simulink model "PID_Throttle"  (R2019b)
settings: Solver=FixedStepDiscrete  StartTime=0.0  StopTime=10.0  RelTol=1e-3
PreLoadFcn:
  | DLRNLPD =1
  | DLRIAMAXA = 1
  | CWDKNOLU = 1
  | DANTGESWNV = 1
  | DLRKPONLP0 = 1
  | DLRKPONLP3 = 1
  | CWDKNOLU = 1
  | DANTGESWNV = 1
  | DLRKPONLP0 = 1
  | DLRKDONLP0 = 1
  | DLRKPUNLP3 = 1
  | DANTSCHWNV = 1
  | DLRUMABAND = 1
  | DLRKDUNLP3 = 1
  | DLRUMAIINI = 1
undefined symbols (not defined in the file): DLRHAFTMN, DLRININI, DLRKREIS
libraries: simulink x3
settings Model: Creator=Guest-Pasand  LastModifiedBy=Guest-Pasand
settings OptimizationCC: DefaultParameterBehavior=Inlined  UseDivisionForNetSlopeComputation=on  GainParamInheritBuiltInType=on  UseFloatMulNetSlope=on  InlineInvariantSignals=on  PassReuseOutputArgsAs=Individual arguments  ZeroExternalMemoryAtStartup=off  ZeroInternalMemoryAtStartup=off  NoFixptDivByZeroProtection=on  EfficientFloat2IntCast=on  LifeSpan=1  OptimizeBlockOrder=speed  DifferentSizesBufferReuse=on  EfficientTunableParamExpr=on
settings DebuggingCC: ParameterTunabilityLossMsg=error
settings HardwareCC: ProdBitPerPointer=32  ProdBitPerSizeT=32  ProdBitPerPtrDiffT=32  ProdLargestAtomicInteger=Long  ProdLargestAtomicFloat=Double  ProdWordSize=32  ProdLongLongMode=on  ProdHWDeviceType=ARM Compatible->ARM Cortex
settings SFSimCC: MATLABDynamicMemAlloc=off
settings RTWCC: SystemTargetFile=ert.tlc  GenCodeOnly=on  TemplateMakefile=ert_default_tmf  GenerateReport=on  IncludeHyperlinkInReport=on  LaunchReport=on  GenerateTraceInfo=on  GenerateTraceReport=on  GenerateTraceReportSl=on  GenerateTraceReportSf=on  GenerateTraceReportEml=on  GenerateCodeMetricsReport=on
settings CodeAppCC: ForceParamTrailComments=on  IgnoreCustomStorageClasses=off  OperatorAnnotations=on  SimulinkDataObjDesc=on  SFDataObjDesc=on  CustomSymbolStrGlobalVar=rt$N$M  CustomSymbolStrType=$N$M  CustomSymbolStrFcn=$N$M$F  CustomSymbolStrMacro=$N$M  InsertBlockDesc=on
settings ERTTargetCC: TargetLangStandard=C99 (ISO)  GenerateSampleERTMain=on  IncludeMdlTerminateFcn=off  CombineSignalStateStructs=on  SuppressErrorStatus=on  SupportAbsoluteTime=off  SupportComplex=off  InlinedParameterPlacement=NonHierarchical  ERTCustomFileTemplate=example_file_process.tlc  ERTFilePackagingFormat=CompactWithDataFile

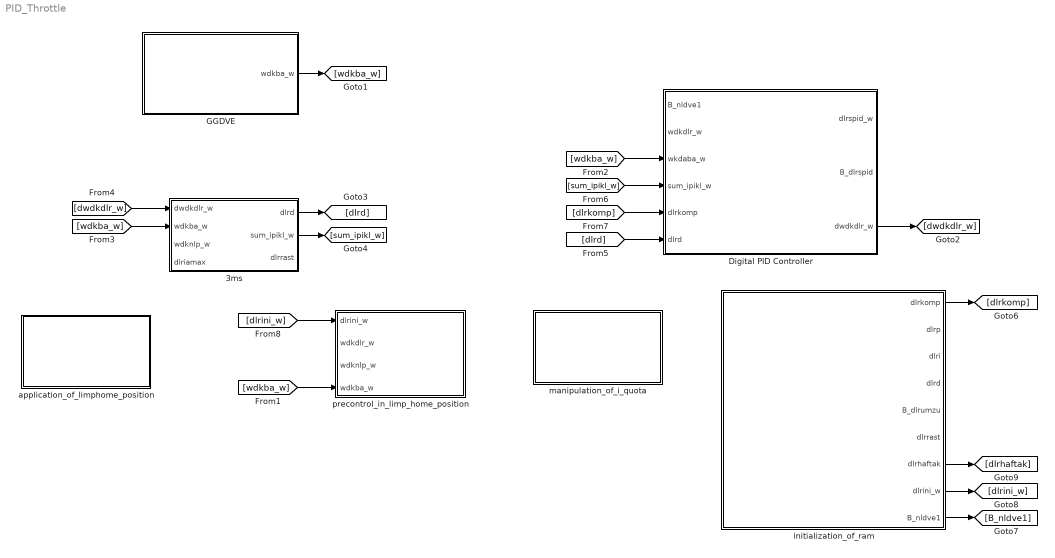
== system PID_Throttle ==
  3ms : Subsystem
  Digital PID Controller : Subsystem
  GGDVE : Subsystem
  application_of_limphome_position : Subsystem
  initialization_of_ram : Subsystem
  "manipulation_of_i_quota " : Subsystem
  precontrol_in_limp_home_position : Subsystem
  wires:
  GGDVE/1(wdkba_w) -> [wdkba_w]
  [wdkba_w] -> precontrol_in_limp_home_position/4(wdkba_w)
  [wdkba_w] -> Digital PID Controller/3(wkdaba_w)
  [wdkba_w] -> 3ms/2(wdkba_w)
  Digital PID Controller/3("dwdkdlr_w ") -> [dwdkdlr_w]
  [dwdkdlr_w] -> 3ms/1(dwdkdlr_w)
  3ms/1(dlrd) -> [dlrd]
  [dlrd] -> Digital PID Controller/6(dlrd)
  [sum_ipikl_w] -> Digital PID Controller/4(sum_ipikl_w)
  3ms/2(sum_ipikl_w) -> [sum_ipikl_w]
  initialization_of_ram/1(dlrkomp) -> [dlrkomp]
  [dlrkomp] -> Digital PID Controller/5(dlrkomp)
  initialization_of_ram/9(B_nldve1) -> [B_nldve1]
  initialization_of_ram/8(dlrini_w) -> [dlrini_w]
  initialization_of_ram/7("dlrhaftak ") -> [dlrhaftak]
  [dlrini_w] -> precontrol_in_limp_home_position/1(dlrini_w)

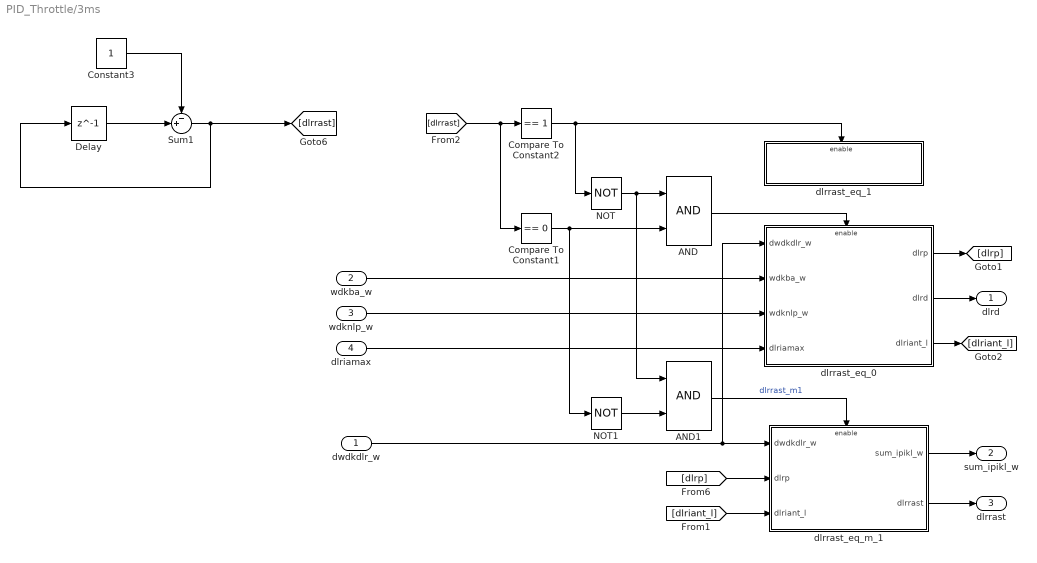
== system PID_Throttle/3ms ==
  dwdkdlr_w : Inport
  wdkba_w : Inport  Port=2
  wdknlp_w : Inport  Port=3
  dlriamax : Inport  Port=4
  AND : Logic  AllPortsSameDT=off  OutDataTypeStr=boolean
  AND1 : Logic  AllPortsSameDT=off  OutDataTypeStr=boolean
  Compare To Constant1 : simulink/Logic and Bit Operations/Compare To Constant  relop===  const=0  OutDataTypeStr=boolean
  Compare To Constant2 : simulink/Logic and Bit Operations/Compare To Constant  relop===  const=1  OutDataTypeStr=boolean
  Constant3 : Constant  VectorParams1D=off  OutDataTypeStr=int8
  Delay : Delay  DelayLength=1  InitialCondition=0
  NOT : Logic  Operator=NOT  IconShape=distinctive  AllPortsSameDT=off  OutDataTypeStr=boolean
  NOT1 : Logic  Operator=NOT  IconShape=distinctive  AllPortsSameDT=off  OutDataTypeStr=boolean
  Sum1 : Sum  Inputs=-+|
  dlrrast_eq_0 : Subsystem
  dlrrast_eq_1 : Subsystem
  dlrrast_eq_m_1 : Subsystem
  dlrd : Outport
  sum_ipikl_w : Outport  Port=2
  dlrrast : Outport  Port=3
  wires:
  Sum1/1 -> Delay/1, [dlrrast]
  Delay/1 -> Sum1/2
  Constant3/1 -> Sum1/1
  Compare To Constant1/1 -> NOT1/1, AND/2
  [dlrrast] -> Compare To Constant1/1, Compare To Constant2/1
  dlrrast_eq_0/1(dlrp) -> [dlrp]
  Compare To Constant2/1 -> dlrrast_eq_1/Enable, NOT/1
  AND/1 -> dlrrast_eq_0/Enable
  NOT/1 -> AND1/1, AND/1
  NOT1/1 -> AND1/2
  AND1/1 -> dlrrast_eq_m_1/Enable  "dlrrast_m1"
  [dlrp] -> dlrrast_eq_m_1/2(dlrp)
  dlrrast_eq_0/3(dlriant_l) -> [dlriant_l]
  [dlriant_l] -> dlrrast_eq_m_1/3(dlriant_l)
  dwdkdlr_w/1 -> dlrrast_eq_m_1/1(dwdkdlr_w), dlrrast_eq_0/1(dwdkdlr_w)
  wdkba_w/1 -> dlrrast_eq_0/2(wdkba_w)
  wdknlp_w/1 -> dlrrast_eq_0/3(wdknlp_w)
  dlrrast_eq_0/2(dlrd) -> dlrd/1
  dlriamax/1 -> dlrrast_eq_0/4(dlriamax)
  dlrrast_eq_m_1/1(sum_ipikl_w) -> sum_ipikl_w/1
  dlrrast_eq_m_1/2(dlrrast) -> dlrrast/1

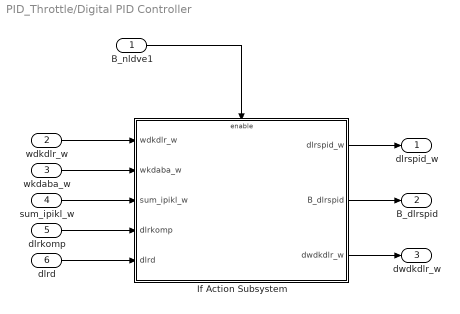
== system PID_Throttle/Digital PID Controller ==
  B_nldve1 : Inport  OutDataTypeStr=boolean
  wdkdlr_w : Inport  Port=2
  wkdaba_w : Inport  Port=3
  sum_ipikl_w : Inport  Port=4
  dlrkomp : Inport  Port=5
  dlrd : Inport  Port=6
  If Action Subsystem : Subsystem  TreatAsAtomicUnit=on
  dlrspid_w : Outport
  B_dlrspid : Outport  Port=2
  "dwdkdlr_w " : Outport  Port=3
  wires:
  wdkdlr_w/1 -> If Action Subsystem/1(wdkdlr_w)
  If Action Subsystem/1(dlrspid_w) -> dlrspid_w/1
  If Action Subsystem/2(B_dlrspid) -> B_dlrspid/1
  B_nldve1/1 -> If Action Subsystem/Enable
  dlrd/1 -> If Action Subsystem/5("dlrd ")
  dlrkomp/1 -> If Action Subsystem/4(dlrkomp)
  sum_ipikl_w/1 -> If Action Subsystem/3(sum_ipikl_w)
  wkdaba_w/1 -> If Action Subsystem/2(wkdaba_w)
  If Action Subsystem/3(dwdkdlr_w) -> "dwdkdlr_w "/1

== system PID_Throttle/GGDVE ==
  wdkba_w : Outport

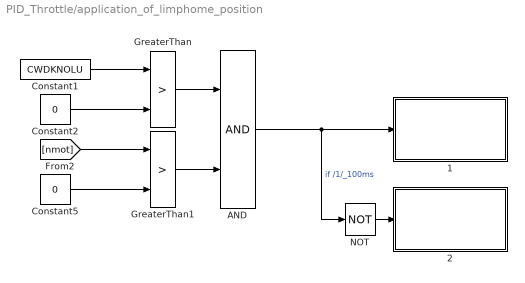
== system PID_Throttle/application_of_limphome_position ==
  1 : Subsystem
  2 : Subsystem
  AND : Logic  AllPortsSameDT=off  OutDataTypeStr=boolean
  Constant1 : Constant  Value=CWDKNOLU  VectorParams1D=off  OutDataTypeStr=int8
  Constant2 : Constant  Value=0  VectorParams1D=off  OutDataTypeStr=int8
  Constant5 : Constant  Value=0  VectorParams1D=off  OutDataTypeStr=int8
  GreaterThan : RelationalOperator  Operator=>  OutDataTypeStr=boolean  RndMeth=Simplest
  GreaterThan1 : RelationalOperator  Operator=>  OutDataTypeStr=boolean  RndMeth=Simplest
  NOT : Logic  Operator=NOT  IconShape=distinctive  AllPortsSameDT=off  OutDataTypeStr=boolean
  wires:
  Constant1/1 -> GreaterThan/1
  Constant2/1 -> GreaterThan/2
  Constant5/1 -> GreaterThan1/2
  [nmot] -> GreaterThan1/1
  GreaterThan/1 -> AND/1
  GreaterThan1/1 -> AND/2
  AND/1 -> NOT/1, 1/Enable  "if /1/_100ms"
  NOT/1 -> 2/Enable

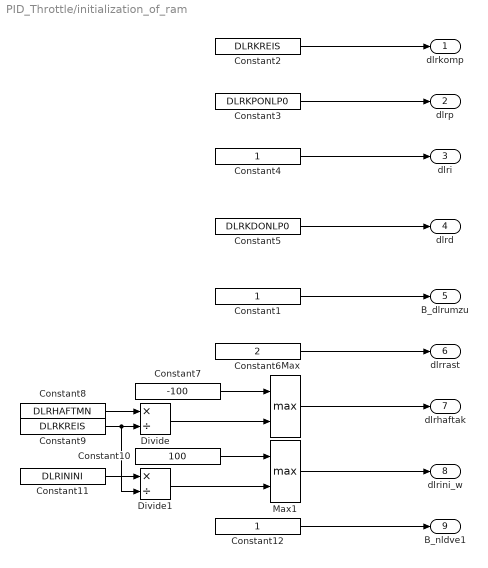
== system PID_Throttle/initialization_of_ram ==
  Constant1 : Constant  VectorParams1D=off
  Constant10 : Constant  Value=100  VectorParams1D=off
  Constant11 : Constant  Value=DLRININI  VectorParams1D=off
  Constant12 : Constant  VectorParams1D=off
  Constant2 : Constant  Value=DLRKREIS  VectorParams1D=off
  Constant3 : Constant  Value=DLRKPONLP0  VectorParams1D=off
  Constant4 : Constant  VectorParams1D=off
  Constant5 : Constant  Value=DLRKDONLP0  VectorParams1D=off
  Constant6 : Constant  Value=2  VectorParams1D=off
  Constant7 : Constant  Value=-100  VectorParams1D=off
  Constant8 : Constant  Value=DLRHAFTMN  VectorParams1D=off
  Constant9 : Constant  Value=DLRKREIS  VectorParams1D=off
  Divide : Product  Inputs=*/
  Divide1 : Product  Inputs=*/
  Max : MinMax  Function=max  Inputs=2
  Max1 : MinMax  Function=max  Inputs=2
  dlrkomp : Outport
  dlrp : Outport  Port=2
  "dlri " : Outport  Port=3
  dlrd : Outport  Port=4
  "B_dlrumzu " : Outport  Port=5
  dlrrast : Outport  Port=6
  "dlrhaftak " : Outport  Port=7
  dlrini_w : Outport  Port=8
  B_nldve1 : Outport  Port=9
  wires:
  Constant2/1 -> dlrkomp/1
  Constant3/1 -> dlrp/1
  Constant4/1 -> "dlri "/1
  Constant5/1 -> dlrd/1
  Constant1/1 -> "B_dlrumzu "/1
  Constant6/1 -> dlrrast/1
  Constant7/1 -> Max/1
  Constant8/1 -> Divide/1
  Divide/1 -> Max/2
  Divide1/1 -> Max1/2
  Constant9/1 -> Divide1/2, Divide/2
  Constant11/1 -> Divide1/1
  Constant10/1 -> Max1/1
  Max/1 -> "dlrhaftak "/1
  Max1/1 -> dlrini_w/1
  Constant12/1 -> B_nldve1/1

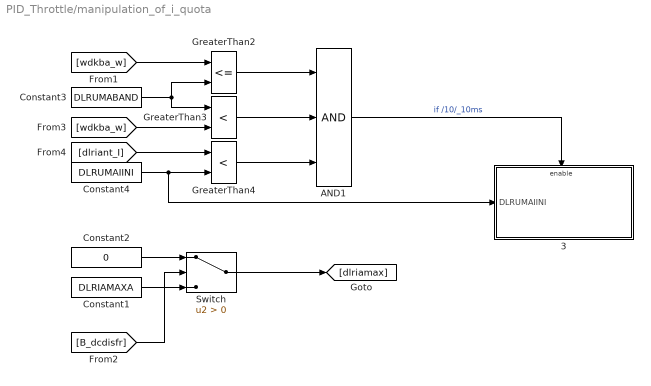
== system PID_Throttle/manipulation_of_i_quota  ==
  3 : Subsystem
  AND1 : Logic  Inputs=3  AllPortsSameDT=off  OutDataTypeStr=boolean
  Constant1 : Constant  Value=DLRIAMAXA  VectorParams1D=off  OutDataTypeStr=int8
  Constant2 : Constant  Value=0  VectorParams1D=off  OutDataTypeStr=int8
  Constant3 : Constant  Value=DLRUMABAND  VectorParams1D=off  OutDataTypeStr=int8
  Constant4 : Constant  Value=DLRUMAIINI  VectorParams1D=off  OutDataTypeStr=int8
  GreaterThan2 : RelationalOperator  Operator=<=  OutDataTypeStr=boolean  RndMeth=Simplest
  GreaterThan3 : RelationalOperator  Operator=<  OutDataTypeStr=boolean  RndMeth=Simplest
  GreaterThan4 : RelationalOperator  Operator=<  OutDataTypeStr=boolean  RndMeth=Simplest
  Switch : Switch  Criteria=u2 > Threshold
  wires:
  [wdkba_w] -> GreaterThan2/1
  Constant3/1 -> GreaterThan2/2, GreaterThan3/1
  [wdkba_w] -> GreaterThan3/2
  [dlriant_I] -> GreaterThan4/1
  Constant4/1 -> 3/1("DLRUMAIINI "), GreaterThan4/2
  GreaterThan4/1 -> AND1/3
  GreaterThan3/1 -> AND1/2
  GreaterThan2/1 -> AND1/1
  AND1/1 -> 3/Enable  "if /10/_10ms"
  Constant2/1 -> Switch/1
  Constant1/1 -> Switch/3
  [B_dcdisfr] -> Switch/2
  Switch/1 -> [dlriamax]

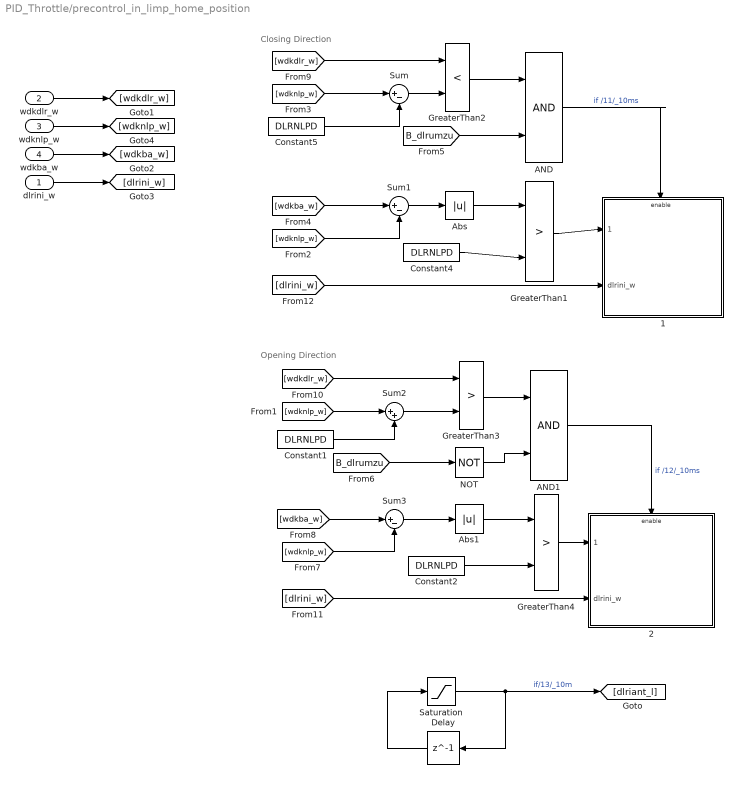
== system PID_Throttle/precontrol_in_limp_home_position ==
  note: Closing Direction
  note: Opening Direction
  dlrini_w : Inport
  wdkdlr_w : Inport  Port=2
  wdknlp_w : Inport  Port=3
  wdkba_w : Inport  Port=4
  1 : Subsystem
  2 : Subsystem
  AND : Logic  AllPortsSameDT=off  OutDataTypeStr=boolean
  AND1 : Logic  AllPortsSameDT=off  OutDataTypeStr=boolean
  Abs : Abs
  Abs1 : Abs
  Constant{1..2,4..5} (4 alike) : Constant  Value=DLRNLPD  VectorParams1D=off  OutDataTypeStr=int8
  Delay : Delay  DelayLength=1
  GreaterThan1 : RelationalOperator  Operator=>  OutDataTypeStr=boolean  RndMeth=Simplest
  GreaterThan2 : RelationalOperator  Operator=<  OutDataTypeStr=boolean  RndMeth=Simplest
  GreaterThan3 : RelationalOperator  Operator=>  OutDataTypeStr=boolean  RndMeth=Simplest
  GreaterThan4 : RelationalOperator  Operator=>  OutDataTypeStr=boolean  RndMeth=Simplest
  NOT : Logic  Operator=NOT  IconShape=distinctive  AllPortsSameDT=off  OutDataTypeStr=boolean
  Saturation : Saturate  UpperLimit=100  LowerLimit=-100
  Sum : Sum  Inputs=|+-
  Sum1 : Sum  Inputs=|+-
  Sum2 : Sum  Inputs=|++
  Sum3 : Sum  Inputs=|+-
  wires:
  Constant5/1 -> Sum/2
  Delay/1 -> Saturation/1
  GreaterThan3/1 -> AND1/1
  [wdkba_w] -> Sum3/1
  Sum3/1 -> Abs1/1
  GreaterThan4/1 -> 2/1(" ")
  Saturation/1 -> [dlriant_l], Delay/1  "if/13/_10m"
  Sum1/1 -> Abs/1
  AND1/1 -> 2/Enable  "if /12/_10ms"
  [wdknlp_w] -> Sum3/2
  Constant2/1 -> GreaterThan4/2
  Abs1/1 -> GreaterThan4/1
  [wdknlp_w] -> Sum2/1
  Constant1/1 -> Sum2/2
  NOT/1 -> AND1/2
  [wdknlp_w] -> Sum1/2
  Sum2/1 -> GreaterThan3/2
  [B_dlrumzu] -> NOT/1
  [wdkba_w] -> Sum1/1
  Sum/1 -> GreaterThan2/2
  Constant4/1 -> GreaterThan1/2
  [wdknlp_w] -> Sum/1
  AND/1 -> 1/Enable  "if /11/_10ms"
  GreaterThan1/1 -> 1/1(" ")
  Abs/1 -> GreaterThan1/1
  [B_dlrumzu] -> AND/2
  GreaterThan2/1 -> AND/1
  wdknlp_w/1 -> [wdknlp_w]
  wdkdlr_w/1 -> [wdkdlr_w]
  wdkba_w/1 -> [wdkba_w]
  [wdkdlr_w] -> GreaterThan2/1
  [wdkdlr_w] -> GreaterThan3/1
  dlrini_w/1 -> [dlrini_w]
  [dlrini_w] -> 2/2(dlrini_w)
  [dlrini_w] -> 1/2(dlrini_w)

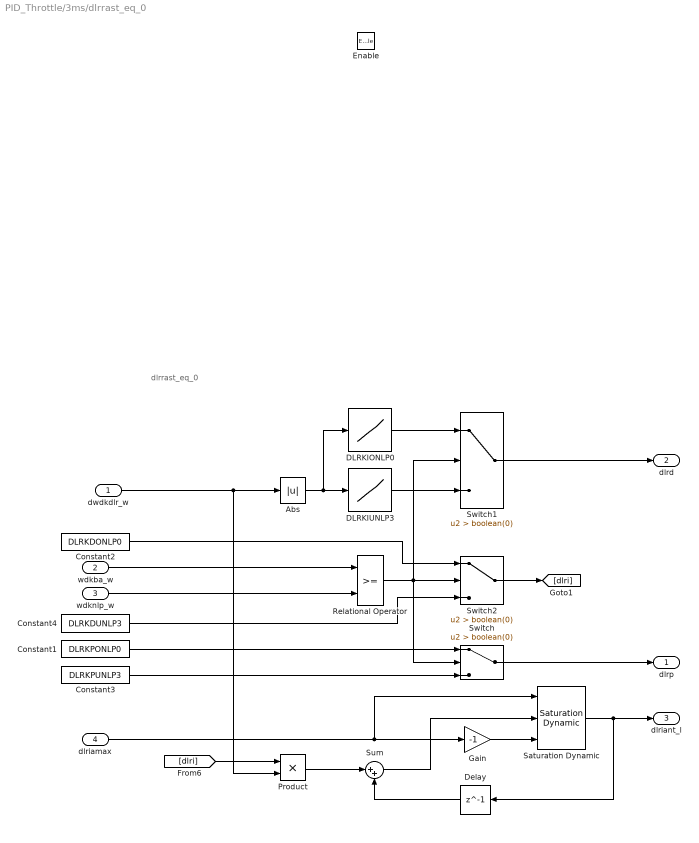
== system PID_Throttle/3ms/dlrrast_eq_0 ==
  note: dlrrast_eq_0
  dwdkdlr_w : Inport
  wdkba_w : Inport  Port=2
  wdknlp_w : Inport  Port=3
  dlriamax : Inport  Port=4
  Enable : EnablePort
  Abs : Abs  ZeroCross=off
  Constant1 : Constant  Value=DLRKPONLP0  VectorParams1D=off  OutDataTypeStr=int8
  Constant2 : Constant  Value=DLRKDONLP0  VectorParams1D=off  OutDataTypeStr=int8
  Constant3 : Constant  Value=DLRKPUNLP3  VectorParams1D=off  OutDataTypeStr=int8
  Constant4 : Constant  Value=DLRKDUNLP3  VectorParams1D=off  OutDataTypeStr=int8
  DLRKIONLP0 : Lookup_n-D  NumberOfTableDimensions=1  BreakpointsForDimension1=[-5:5]  Table=tanh([-5:5])  InternalRulePriority=Speed  RndMeth=Simplest  InputSameDT=on
  DLRKIUNLP3 : Lookup_n-D  NumberOfTableDimensions=1  BreakpointsForDimension1=[-5:5]  Table=tanh([-5:5])  InternalRulePriority=Speed  RndMeth=Simplest  InputSameDT=on
  Delay : Delay  DelayLength=1  InitialCondition=0
  Gain : Gain  Gain=-1  ParamDataTypeStr=double
  Product : Product
  Relational Operator : RelationalOperator  OutDataTypeStr=boolean  RndMeth=Simplest
  Saturation Dynamic : simulink/Discontinuities/Saturation Dynamic  OutMin=[]  OutMax=[]  OutDataTypeStr=Inherit: Same as second input  OutDataType=fixdt(1, 16)  OutScaling=2^-10  DoSatur=off
  Sum : Sum  Inputs=|++
  Switch : Switch  Criteria=u2 > Threshold  Threshold=boolean(0)
  Switch1 : Switch  Criteria=u2 > Threshold  Threshold=boolean(0)
  Switch2 : Switch  Criteria=u2 > Threshold  Threshold=boolean(0)
  dlrp : Outport
  dlrd : Outport  Port=2
  dlriant_l : Outport  Port=3
  wires:
  Switch1/1 -> dlrd/1
  Switch/1 -> dlrp/1
  Saturation Dynamic/1 -> dlriant_l/1, Delay/1
  Constant4/1 -> Switch2/3
  Constant1/1 -> Switch/1
  Constant3/1 -> Switch/3
  Constant2/1 -> Switch2/1
  wdknlp_w/1 -> Relational Operator/2
  Gain/1 -> Saturation Dynamic/3
  Abs/1 -> DLRKIUNLP3/1, DLRKIONLP0/1
  Delay/1 -> Sum/2
  Product/1 -> Sum/1
  Sum/1 -> Saturation Dynamic/2
  dlriamax/1 -> Saturation Dynamic/1, Gain/1
  [dlri] -> Product/1
  DLRKIUNLP3/1 -> Switch1/3
  wdkba_w/1 -> Relational Operator/1
  dwdkdlr_w/1 -> Product/2, Abs/1
  Relational Operator/1 -> Switch1/2, Switch2/2, Switch/2
  DLRKIONLP0/1 -> Switch1/1
  Switch2/1 -> [dlri]

== system PID_Throttle/3ms/dlrrast_eq_1 ==
  Enable : EnablePort

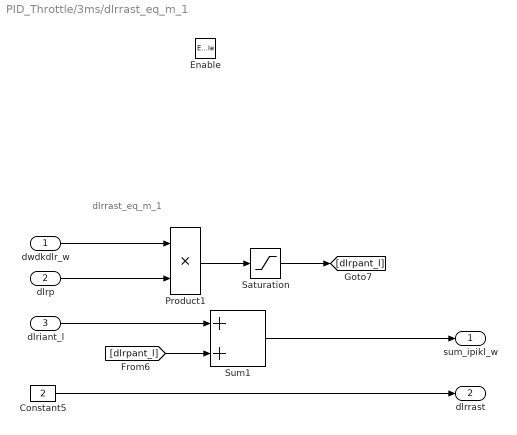
== system PID_Throttle/3ms/dlrrast_eq_m_1 ==
  note: dlrrast_eq_m_1
  dwdkdlr_w : Inport
  dlrp : Inport  Port=2
  dlriant_l : Inport  Port=3
  Enable : EnablePort
  Constant5 : Constant  Value=2  VectorParams1D=off  OutDataTypeStr=int8
  Product1 : Product
  Saturation : Saturate  UpperLimit=800  LowerLimit=800
  Sum1 : Sum
  sum_ipikl_w : Outport
  dlrrast : Outport  Port=2
  wires:
  Constant5/1 -> dlrrast/1
  Sum1/1 -> sum_ipikl_w/1
  Saturation/1 -> [dlrpant_l]
  Product1/1 -> Saturation/1
  dwdkdlr_w/1 -> Product1/1
  dlriant_l/1 -> Sum1/1
  [dlrpant_l] -> Sum1/2
  dlrp/1 -> Product1/2

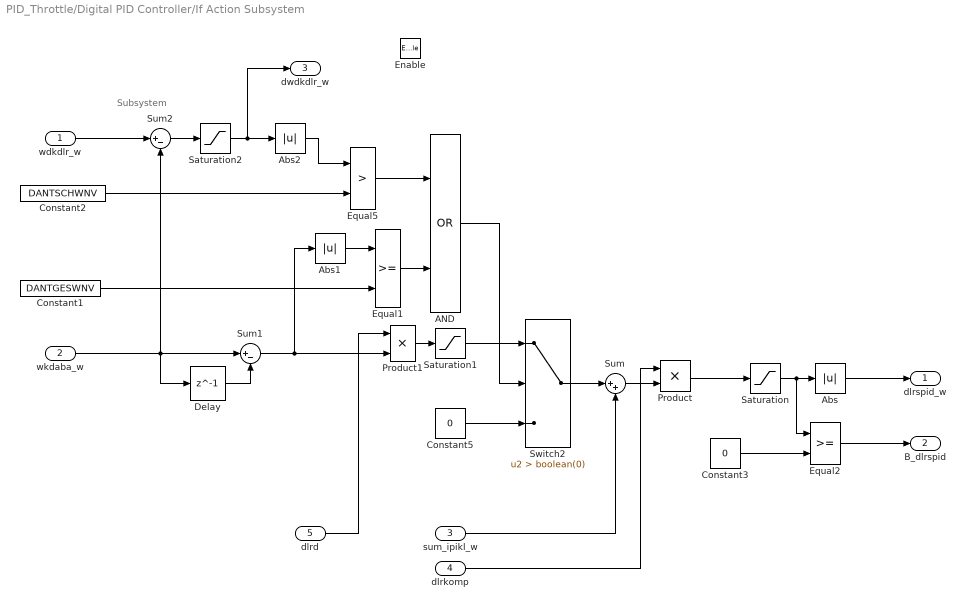
== system PID_Throttle/Digital PID Controller/If Action Subsystem ==
  note: Subsystem
  wdkdlr_w : Inport
  wkdaba_w : Inport  Port=2
  sum_ipikl_w : Inport  Port=3
  dlrkomp : Inport  Port=4
  "dlrd " : Inport  Port=5
  Enable : EnablePort
  AND : Logic  Operator=OR  AllPortsSameDT=off  OutDataTypeStr=boolean
  Abs : Abs  ZeroCross=off
  Abs1 : Abs  ZeroCross=off
  Abs2 : Abs  ZeroCross=off
  Constant1 : Constant  Value=DANTGESWNV  VectorParams1D=off
  Constant2 : Constant  Value=DANTSCHWNV  VectorParams1D=off
  Constant3 : Constant  Value=0  VectorParams1D=off  OutDataTypeStr=int8
  Constant5 : Constant  Value=0  VectorParams1D=off  OutDataTypeStr=uint8
  Delay : Delay  DelayLength=1  InitialCondition=0
  Equal1 : RelationalOperator  OutDataTypeStr=boolean  RndMeth=Simplest
  Equal2 : RelationalOperator  OutDataTypeStr=boolean  ZeroCross=off  RndMeth=Simplest
  Equal5 : RelationalOperator  Operator=>  OutDataTypeStr=boolean  RndMeth=Simplest
  Product : Product
  Product1 : Product
  Saturation : Saturate  UpperLimit=100  LowerLimit=-100  ZeroCross=off
  Saturation1 : Saturate  UpperLimit=1000  LowerLimit=-1000  ZeroCross=off
  Saturation2 : Saturate  UpperLimit=100  LowerLimit=-100  LinearizeAsGain=off  ZeroCross=off
  Sum : Sum  Inputs=|++
  Sum1 : Sum  Inputs=|+-
  Sum2 : Sum  Inputs=|+-
  Switch2 : Switch  Criteria=u2 > Threshold  Threshold=boolean(0)  ZeroCross=off
  dlrspid_w : Outport
  B_dlrspid : Outport  Port=2
  dwdkdlr_w : Outport  Port=3
  wires:
  Product1/1 -> Saturation1/1
  "dlrd "/1 -> Product1/1
  Sum/1 -> Product/2
  Constant1/1 -> Equal1/2
  Constant2/1 -> Equal5/2
  Constant3/1 -> Equal2/2
  Product/1 -> Saturation/1
  Abs1/1 -> Equal1/1
  AND/1 -> Switch2/2
  Delay/1 -> Sum1/2
  Abs2/1 -> Equal5/1
  Saturation1/1 -> Switch2/1
  Saturation/1 -> Equal2/1, Abs/1
  dlrkomp/1 -> Product/1
  sum_ipikl_w/1 -> Sum/2
  Sum1/1 -> Abs1/1, Product1/2
  Constant5/1 -> Switch2/3
  Switch2/1 -> Sum/1
  wdkdlr_w/1 -> Sum2/1
  Saturation2/1 -> dwdkdlr_w/1, Abs2/1
  Sum2/1 -> Saturation2/1
  Equal5/1 -> AND/1
  wkdaba_w/1 -> Delay/1, Sum1/1, Sum2/2
  Equal1/1 -> AND/2
  Equal2/1 -> B_dlrspid/1
  Abs/1 -> dlrspid_w/1

== system PID_Throttle/application_of_limphome_position/1 ==
  Enable : EnablePort
  1 : Subsystem
  Constant2 : Constant  Value=0  VectorParams1D=off  OutDataTypeStr=boolean
  Equal : RelationalOperator  Operator===  OutDataTypeStr=boolean  RndMeth=Simplest
  wires:
  [B_appnolu] -> Equal/1
  Constant2/1 -> Equal/2
  Equal/1 -> 1/Enable  "if /1/"

== system PID_Throttle/application_of_limphome_position/2 ==
  Enable : EnablePort
  Constant2 : Constant  Value=0  VectorParams1D=off  OutDataTypeStr=boolean
  wires:
  Constant2/1 -> [B_appnolu], [B_apnoluv]

== system PID_Throttle/manipulation_of_i_quota /3 ==
  "DLRUMAIINI " : Inport
  Enable : EnablePort
  wires:
  "DLRUMAIINI "/1 -> [dlriant_l]

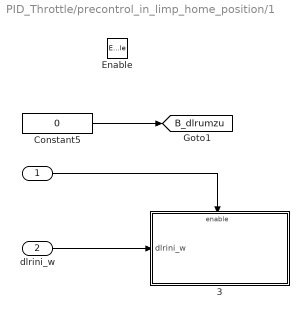
== system PID_Throttle/precontrol_in_limp_home_position/1 ==
  " " : Inport
  dlrini_w : Inport  Port=2
  Enable : EnablePort
  3 : Subsystem
  Constant5 : Constant  Value=0  VectorParams1D=off  OutDataTypeStr=int8
  tag scope: B_dlrumzu=global
  wires:
  " "/1 -> 3/Enable
  Constant5/1 -> [B_dlrumzu]
  dlrini_w/1 -> 3/1("dlrini_w ")

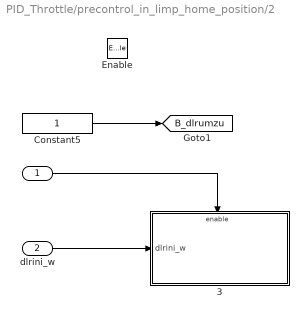
== system PID_Throttle/precontrol_in_limp_home_position/2 ==
  " " : Inport
  dlrini_w : Inport  Port=2
  Enable : EnablePort
  3 : Subsystem
  Constant5 : Constant  VectorParams1D=off  OutDataTypeStr=int8
  tag scope: B_dlrumzu=global
  wires:
  dlrini_w/1 -> 3/1("dlrini_w ")
  Constant5/1 -> [B_dlrumzu]
  " "/1 -> 3/Enable

== system PID_Throttle/application_of_limphome_position/1/1 ==
  Enable : EnablePort
  Constant2 : Constant  VectorParams1D=off  OutDataTypeStr=boolean
  wires:
  Constant2/1 -> [B_apnoluv], [B_appnolu]

== system PID_Throttle/precontrol_in_limp_home_position/1/3 ==
  "dlrini_w " : Inport
  Enable : EnablePort
  Delay : Delay  DelayLength=1
  Sum : Sum  Inputs=|+-
  wires:
  Sum/1 -> Delay/1, [dlriant_l]
  "dlrini_w "/1 -> Sum/1
  Delay/1 -> Sum/2

== system PID_Throttle/precontrol_in_limp_home_position/2/3 ==
  "dlrini_w " : Inport
  Enable : EnablePort
  Delay : Delay  DelayLength=1
  Sum : Sum  Inputs=|++
  wires:
  Delay/1 -> Sum/2
  "dlrini_w "/1 -> Sum/1
  Sum/1 -> [dlriant_l], Delay/1
